simulink model "LKAS_AutoSave_DF_20220421_1805_SW62"  (R2018b)
settings: Solver=FixedStepDiscrete  StartTime=0.0  StopTime=10.0  FixedStep=0.01  RelTol=1e-3
model workspace (MAT data in the model file):
  MCOS : class17 (value not decoded)
  MCOS : class17 (value not decoded)
  MCOS : class17 (value not decoded)
  MCOS : class17 (value not decoded)
  MCOS : class17 (value not decoded)
  MCOS : class17 (value not decoded)
  MCOS : class17 (value not decoded)
  MCOS : class17 (value not decoded)
  MCOS : class17 (value not decoded)
  MCOS : class17 (value not decoded)
  MCOS : class17 (value not decoded)
  MCOS : class17 (value not decoded)
  MCOS : class17 (value not decoded)
  MCOS : class17 (value not decoded)
  MCOS : class17 (value not decoded)
  MCOS : class17 (value not decoded)
  MCOS : class17 (value not decoded)
  MCOS : class17 (value not decoded)
  MCOS : class17 (value not decoded)
  MCOS : class17 (value not decoded)
  MCOS : class17 (value not decoded)
  MCOS : class17 (value not decoded)
  MCOS : class17 (value not decoded)
  MCOS : class17 (value not decoded)
  MCOS : class17 (value not decoded)
  MCOS : class17 (value not decoded)
  MCOS : class17 (value not decoded)
  MCOS : class17 (value not decoded)
  MCOS : class17 (value not decoded)
  MCOS : class17 (value not decoded)
  MCOS : class17 (value not decoded)
  MCOS : class17 (value not decoded)
  MCOS : class17 (value not decoded)
  MCOS : class17 (value not decoded)
  MCOS : class17 (value not decoded)
  MCOS : class17 (value not decoded)
  MCOS : class17 (value not decoded)
  MCOS : class17 (value not decoded)
  MCOS : class17 (value not decoded)
  MCOS : class17 (value not decoded)
  MCOS : class17 (value not decoded)
  MCOS : class17 (value not decoded)
  MCOS : class17 (value not decoded)
  MCOS : class17 (value not decoded)
  MCOS : class17 (value not decoded)
  MCOS : class17 (value not decoded)
  MCOS : class17 (value not decoded)
  MCOS : class17 (value not decoded)
  MCOS : class17 (value not decoded)
  MCOS : class17 (value not decoded)
  MCOS : class17 (value not decoded)
  MCOS : class17 (value not decoded)
  MCOS : class17 (value not decoded)
  MCOS : class17 (value not decoded)
  MCOS : class17 (value not decoded)
  MCOS : class17 (value not decoded)
  MCOS : class17 (value not decoded)
  MCOS : class17 (value not decoded)
  MCOS : class17 (value not decoded)
  MCOS : class17 (value not decoded)
  MCOS : class17 (value not decoded)
  MCOS : class17 (value not decoded)
  MCOS : class17 (value not decoded)
  MCOS : class17 (value not decoded)
  MCOS : class17 (value not decoded)
  MCOS : class17 (value not decoded)
  MCOS : class17 (value not decoded)
  MCOS : class17 (value not decoded)
  MCOS : class17 (value not decoded)
  MCOS : class17 (value not decoded)
  MCOS : class17 (value not decoded)
  MCOS : class17 (value not decoded)
  MCOS : class17 (value not decoded)
  MCOS : class17 (value not decoded)
  MCOS : class17 (value not decoded)
  MCOS : class17 (value not decoded)
  MCOS : class17 (value not decoded)
  MCOS : class17 (value not decoded)
  MCOS : class17 (value not decoded)
  MCOS : class17 (value not decoded)
  MCOS : class17 (value not decoded)
  MCOS : class17 (value not decoded)
  MCOS : class17 (value not decoded)
  MCOS : class17 (value not decoded)
  MCOS : class17 (value not decoded)
  MCOS : class17 (value not decoded)
  MCOS : class17 (value not decoded)
  MCOS : class17 (value not decoded)
  MCOS : class17 (value not decoded)
  MCOS : class17 (value not decoded)
  MCOS : class17 (value not decoded)
  MCOS : class17 (value not decoded)
  MCOS : class17 (value not decoded)
  MCOS : class17 (value not decoded)
  MCOS : class17 (value not decoded)
  MCOS : class17 (value not decoded)
  MCOS : class17 (value not decoded)
  MCOS : class17 (value not decoded)
  MCOS : class17 (value not decoded)
  MCOS : class17 (value not decoded)
  MCOS : class17 (value not decoded)
  MCOS : class17 (value not decoded)
  MCOS : class17 (value not decoded)
  MCOS : class17 (value not decoded)
  MCOS : class17 (value not decoded)
  MCOS : class17 (value not decoded)
  MCOS : class17 (value not decoded)
  MCOS : class17 (value not decoded)
  MCOS : class17 (value not decoded)
  MCOS : class17 (value not decoded)
undefined symbols (not defined in the file): LKA_CarWidth, LKA_SampleTime, LKA_StrRatio_C, LKA_Veh2CamL_C, LKA_Veh2CamW_C, LKA_WhlBaseL_C, LL_CompHdAg_C, LL_CompSWA_C, LL_CrvtPrvwT_C, LL_DesDvt_C, LL_DvtComp_C, LL_DvtPrvwT_C, LL_DvtSpdDet_vDvtSpdMin_C, LL_HandsOff_ExitTime, LL_HandsOff_TextTime, LL_HandsOff_WarnTime, LL_HdAgExT_C, LL_HdAgPrvwT_C, LL_LAccMax_C, LL_LAccRMax_C, LL_LDW_EarliestWarnLine_C, LL_LDW_LatestWarnLine_C, LL_LDWS_SUPPRESS_HEADING, LL_LFClb_TFC_FfCtlRatio_C, LL_LFClb_TFC_KdBalance_C, LL_LFClb_TFC_KdMaxSWA_C, LL_LFClb_TFC_KdV1_C, LL_LFClb_TFC_KdV2_C, LL_LFClb_TFC_KdVehSpdLwr_C, LL_LFClb_TFC_KdVehSpdUpr_C, LL_LFClb_TFC_Ki_C, LL_LFClb_TFC_KiMaxSWA_C, LL_LFClb_TFC_Kp_C, LL_LFClb_TFC_KpKlat_C, LL_LFClb_TFC_KpV1_C, LL_LFClb_TFC_KpV2_C, LL_LFClb_TFC_KpVehSpdLwr_C, LL_LFClb_TFC_KpVehSpdUpr_C, LL_LFClb_TFC_PrvwT_C, LL_LKA_EarliestWarnLine_C, LL_LKA_EnableLine_DvtMax, LL_LKA_EnableLine_DvtMin, LL_LKA_EnableLine_Max, LL_LKA_LatestWarnLine_C, LL_LKAExPrcs_ExitC0Dvt, LL_LKAExPrcs_ExitC0Swt, LL_LKAExPrcs_tiExitDelayTime3, LL_LKAExPrcs_tiExitTime1, LL_LKAExPrcs_tiExitTime2, LL_LKAExPrcs_tiExitTime3, LL_LKAS_OUT_OF_CONTROL_LAT_VEL, LL_LKAS_OUT_OF_CONTROL_TTLC, LL_LKASWASyn_M0, LL_LKASWASyn_M1, LL_LKASWASyn_M2, LL_LKASWASyn_M3D, LL_LKASWASyn_M3K_DT, LL_LKASWASyn_M3K_MSD, LL_LKASWASyn_M4K, LL_LKASWASyn_SWAaddMax ... (+51)
libraries: simulink x241, canmsglib x6, dspstat3 x3, simulink_extras x1
(part 6 of 18)

== system LKAS_AutoSave_DF_20220421_1805_SW62/LKAS/LL/LLOn/LKA Input Processing (LKAInP) ==
  bsInInfo : Inport
  bsLLClb : Inport  Port=2
  ActFlg : Inport  Port=3
  Bus Creator2 : BusCreator  Inputs=10
  Curvature Calculation (Crvt) : Subsystem
  Delay : Delay  DelayLength=1
  Deviation Calculation (Dvt) : Subsystem
  Heading Angle Calculation (HdAg) : Subsystem
  Lane Width Calculation (LW) : Subsystem
  Previewed Curvature Calculation (PrCrvt) : Subsystem
  Previewed Deviation Calculation (PrDvt) : Subsystem
  Previewed Heading Angle Calculation (PrHdAg) : Subsystem
  Steering Wheel Position Calculation (SWAPosCal) : Subsystem
  TTLC Calculation (TTLCCalc) : Subsystem  Description=|
      | Block Name: TTLC Calculation
      | Ab.: TTLCCalc
      | No.: 1.1.1.1
      | Rev: 0.0.1
      | Update Date: 19-3-26
  Under The Limit (UndrLim) : Subsystem
  bsLKAInPInfo : Outport
  wires:
  [bsTTLCInfo] -> Previewed Heading Angle Calculation (PrHdAg)/3(PrHdAg_bsTTLCInfo)  "bsTTLCInfo"
  TTLC Calculation (TTLCCalc)/1(TTLCCalc_bsTTLCInfo) -> [bsTTLCInfo]  "bsTTLCInfo"
  Previewed Deviation Calculation (PrDvt)/1(PrvwDvt_bsPrvwDvtInfo) -> [bsPrDvtInfo]  "bsPrDvtInfo"
  Previewed Heading Angle Calculation (PrHdAg)/1(PrHdAg_bsPrHdAgInfo) -> [bsPrHdAgInfo]  "bsPrHdAgInfo"
  [bsPrCrvtInfo] -> TTLC Calculation (TTLCCalc)/4(TTLCCalc_bsPrCrvtInfo)  "bsPrCrvtInfo"
  Previewed Curvature Calculation (PrCrvt)/1(PrvwCrvt_bsPrvwCrvtInfo) -> [bsPrCrvtInfo]  "bsPrCrvtInfo"
  [bsDvtInfo] -> TTLC Calculation (TTLCCalc)/1(TTLCCalc_bsDvtInfo)  "bsDvtInfo"
  Deviation Calculation (Dvt)/1(Dvt_bsDvtInfo) -> [bsDvtInfo]  "bsDvtInfo"
  [bsHdAgInfo] -> TTLC Calculation (TTLCCalc)/5(TTLCCalc_bsHdAgInfo)  "bsHdAgInfo"
  Heading Angle Calculation (HdAg)/1(HdAg_bsHdAgInfo) -> [bsHdAgInfo]  "bsHdAgInfo"
  Curvature Calculation (Crvt)/1(Crvt_bsCrvtInfo) -> [bsCrvtInfo]  "bsCrvtInfo"
  Under The Limit (UndrLim)/1(UndrLim_bsUndrLimInfo) -> [bsUndrLimInfo]  "bsUndrLimInfo"
  Steering Wheel Position Calculation (SWAPosCal)/1(SWAPosCal) -> [phiSWAPos]  "phiSWAPos"
  Lane Width Calculation (LW)/1(LW_LaneWidth) -> [LaneWidth]  "LaneWidth"
  Delay/1 -> Previewed Curvature Calculation (PrCrvt)/3(PrvwCrvt_stLKAActvFlg)
  ActFlg/1 -> Delay/1
  Bus Creator2/1 -> bsLKAInPInfo/1
  [bsPrCrvtInfo] -> Bus Creator2/7  "bsPrCrvtInfo"
  [bsPrDvtInfo] -> Bus Creator2/9  "bsPrDvtInfo"
  [bsCrvtInfo] -> Bus Creator2/4  "bsCrvtInfo"
  [bsDvtInfo] -> Bus Creator2/6  "bsDvtInfo"
  [bsUndrLimInfo] -> Bus Creator2/3  "bsUndrLimInfo"
  [phiSWAPos] -> Bus Creator2/2  "phiSWAPos"
  [LaneWidth] -> Bus Creator2/1  "LaneWidth"
  [bsTTLCInfo] -> Bus Creator2/10  "bsTTLCInfo"
  [bsPrHdAgInfo] -> Bus Creator2/8  "bsPrHdAgInfo"
  bsLLClb/1 -> TTLC Calculation (TTLCCalc)/2(TTLCCalc_bsLLClb), Previewed Curvature Calculation (PrCrvt)/2(PrvwCrvt_tiCrvtPrvwT_C), Steering Wheel Position Calculation (SWAPosCal)/2(SWAPosCal_bsLLClb), Under The Limit (UndrLim)/2(UndrLim_bsLLClb), Deviation Calculation (Dvt)/2(Dvt_bsLLClb), Previewed Heading Angle Calculation (PrHdAg)/2(PrHdAg_bsLLClb), Previewed Deviation Calculation (PrDvt)/1(PrdcDvt_bsLLClb)
  [bsHdAgInfo] -> Bus Creator2/5  "bsHdAgInfo"
  bsInInfo/1 -> Steering Wheel Position Calculation (SWAPosCal)/1(SWAPosCal_bsInInfoSyn), Lane Width Calculation (LW)/1(LW_bsInInfoSyn), Under The Limit (UndrLim)/1(UndrLim_bsInInfoSyn), Curvature Calculation (Crvt)/1(PrvwCrvt_bsInInfoSyn), Heading Angle Calculation (HdAg)/1(HdAg_bsInInfoSyn), Deviation Calculation (Dvt)/1(Dvt_bsInInfoSyn), Previewed Curvature Calculation (PrCrvt)/1(PrvwCrvt_bsInInfoSyn), Previewed Deviation Calculation (PrDvt)/2(PrvwDvt_bsInInfoSyn), TTLC Calculation (TTLCCalc)/3(TTLCCalc_bsInfo), Previewed Heading Angle Calculation (PrHdAg)/1(PrHdAg_bsInInfoSyn)

== system LKAS_AutoSave_DF_20220421_1805_SW62/LKAS/LL/LLOn/LL State Determination (LLStateDet) ==
  bsInInfo : Inport
  bsLKAInPInfo : Inport  Port=2
  bsLLClb : Inport  Port=3
  ExitFlg : Inport  Port=4
  bsSignalFault : Inport  Port=5
  Bus Creator : BusCreator  Inputs=3
  Delay : Delay  DelayLength=1
  Delay1 : Delay  DelayLength=1
  LDW_State_Machine : Stateflow chart  Description=|  TreatAsAtomicUnit=on
      | Block Name: LDW State Machine
      | Ab.: LDWSM
      | No.: 1.1.2.0
      | Rev: 0.0.1
      | Update Date: 19-3-26
      settings: RTWSystemCode=Nonreusable function
  LKA_State_Machine : Stateflow chart  Description=|  TreatAsAtomicUnit=on
      | Block Name: LKA State Machine
      | Ab.: LKASM
      | No.: 1.1.3.0
      | Rev: 0.0.1
      | Update Date: 19-3-26
      settings: RTWSystemCode=Nonreusable function
  LL State Machine Conditions (LLSMCon) : Subsystem
  bsLLState : Outport
  stLDWActvFlg : Outport  Port=2
  stLKAActvFlg : Outport  Port=3
  Disable_Reason : Outport  Port=4
  Fault_Reason : Outport  Port=5
  tag scope: LDW_State_Mon=global, LKA_State_Mon=global
  wires:
  [LKA_Mode] -> Bus Creator/2
  [LKA_Mode] -> LKA_State_Machine/1(LKA_Mode)
  [LKA_Mode] -> LDW_State_Machine/1(LKA_Mode)
  LL State Machine Conditions (LLSMCon)/1(LKA_Mode) -> [LKA_Mode]  "LKA_Mode"
  LL State Machine Conditions (LLSMCon)/13(Fault_Reason) -> Fault_Reason/1
  LL State Machine Conditions (LLSMCon)/12(Disable_Reason) -> Disable_Reason/1
  bsSignalFault/1 -> LL State Machine Conditions (LLSMCon)/6(bsSignalFault)
  Delay/1 -> LL State Machine Conditions (LLSMCon)/5(ExitFlg)
  bsLLClb/1 -> LL State Machine Conditions (LLSMCon)/3(bsLLClb)
  ExitFlg/1 -> Delay/1
  bsLKAInPInfo/1 -> LL State Machine Conditions (LLSMCon)/2(bsLKAInPInfo)
  bsInInfo/1 -> LL State Machine Conditions (LLSMCon)/1(bsInInfo)
  LL State Machine Conditions (LLSMCon)/11(LKA_Fault) -> LKA_State_Machine/6(LKA_Fault)
  LL State Machine Conditions (LLSMCon)/10(stLKADeactvCSyn) -> LKA_State_Machine/5(stLKADeactvCSyn)
  LL State Machine Conditions (LLSMCon)/9(stLKAActvCSyn) -> LKA_State_Machine/4(stLKAActvCSyn)
  LL State Machine Conditions (LLSMCon)/8(stLKADisblCSyn) -> LKA_State_Machine/3(stLKADisblCSyn)
  LL State Machine Conditions (LLSMCon)/7(stLKAEnaCSyn) -> LKA_State_Machine/2(stLKAEnaCSyn)
  LL State Machine Conditions (LLSMCon)/6(LDW_Fault) -> LDW_State_Machine/6(LDW_Fault)
  LDW_State_Machine/2(stLDWState) -> Bus Creator/1, [LDW_State_Mon]  "LDW_State"
  LKA_State_Machine/2(stLKAState) -> [LKA_State_Mon], Bus Creator/3  "LKA_State"
  Bus Creator/1 -> Delay1/1, bsLLState/1  "bsLLState"
  Delay1/1 -> LL State Machine Conditions (LLSMCon)/4(bsLLState)
  LKA_State_Machine/1(stLKAActvFlg) -> stLKAActvFlg/1
  LDW_State_Machine/1(stLDWActvFlg) -> stLDWActvFlg/1
  LL State Machine Conditions (LLSMCon)/5(stLDWDeactvCSyn) -> LDW_State_Machine/5(stLDWDeactvCSyn)  "stLDWDeactvCSyn"
  LL State Machine Conditions (LLSMCon)/4(stLDWActvCSyn) -> LDW_State_Machine/4(stLDWActvCSyn)
  LL State Machine Conditions (LLSMCon)/3(stLDWDisblCSyn) -> LDW_State_Machine/3(stLDWDisblCSyn)
  LL State Machine Conditions (LLSMCon)/2(stLDWEnaCSyn) -> LDW_State_Machine/2(stLDWEnaCSyn)

== system LKAS_AutoSave_DF_20220421_1805_SW62/LKAS/LL/LLOn/LL_Mon ==
  Disable_Reason : Inport
  Fault_Reason : Inport  Port=2
  LKAMon : Inport  Port=3
  Bus : BusCreator  Inputs=5
  BusInP : BusCreator  Inputs=2
  BusState : BusCreator  Inputs=2
  LLMon : Outport
  wires:
  Fault_Reason/1 -> Bus/5  "Fault_Reason"
  Disable_Reason/1 -> Bus/4  "Disable_Reason"
  BusState/1 -> [StateMon]  "StateMon"
  BusInP/1 -> [InPMon]  "InPMon"
  [LKA_State_Mon] -> BusState/2  "LKA_State_Mon"
  [LDW_State_Mon] -> BusState/1  "LDW_State_Mon"
  [RGTTTLC_Mon] -> BusInP/2  "RGTTTLC_Mon"
  [LFTTTLC_Mon] -> BusInP/1  "LFTTTLC_Mon"
  Bus/1 -> LLMon/1  "LLMon"
  LKAMon/1 -> Bus/3
  [StateMon] -> Bus/2
  [InPMon] -> Bus/1

== system LKAS_AutoSave_DF_20220421_1805_SW62/LKAS/LL/LLOut/Angle2Trq ==
  LKA_Torque_Req : Inport
  Target_Angle : Inport  Port=2
  Stearing_Angle : Inport  Port=3
  Constant : Constant  Value=5  OutDataTypeStr=single
  Constant1 : Constant  Value=-5  OutDataTypeStr=single
  Constant3 : Constant  Value=5  OutDataTypeStr=single
  Constant4 : Constant  Value=-5  OutDataTypeStr=single
  Rate Limiter Dynamic : Subsystem
  Saturation Dynamic : Subsystem
  Subsystem : Subsystem
  torque : Outport  OutputWhenDisabled=reset  InitialOutput=0
  wires:
  LKA_Torque_Req/1 -> Subsystem/Enable  "LKA_Torque_Req"
  Subsystem/1(in_trq) -> Rate Limiter Dynamic/2(u)  "in_trq"
  Stearing_Angle/1 -> Subsystem/2(Stearing_Angle)  "Stearing_Angle"
  Target_Angle/1 -> Subsystem/1(Target_Angle)  "Target_Angle"
  Constant/1 -> Rate Limiter Dynamic/1(up)
  Constant1/1 -> Rate Limiter Dynamic/3(lo)
  Rate Limiter Dynamic/1(Y) -> Saturation Dynamic/2(u)  "RL_trq"
  Constant3/1 -> Saturation Dynamic/1(up)
  Constant4/1 -> Saturation Dynamic/3(lo)
  Saturation Dynamic/1(y) -> torque/1  "Saturation_trq"

== system LKAS_AutoSave_DF_20220421_1805_SW62/LKAS/LLClb/LLSMConClb/ICv to v10 ==
  In1 : Inport
  Add : Sum  Inputs=+-
  Constant : Constant  Value=2.5  OutDataTypeStr=single
  Gain : Gain  Gain=1/1.02
  Out1 : Outport
  wires:
  Gain/1 -> Out1/1
  Constant/1 -> Add/2
  Add/1 -> Gain/1
  In1/1 -> Add/1

== system LKAS_AutoSave_DF_20220421_1805_SW62/LKAS/LLClb/LLSMConClb/ICv to v11 ==
  In1 : Inport
  Add : Sum  Inputs=+-
  Constant : Constant  Value=2.5  OutDataTypeStr=single
  Gain : Gain  Gain=1/1.02
  Out1 : Outport
  wires:
  In1/1 -> Add/1
  Add/1 -> Gain/1
  Constant/1 -> Add/2
  Gain/1 -> Out1/1

== system LKAS_AutoSave_DF_20220421_1805_SW62/LKAS/LLClb/LLSMConClb/ICv to v6 ==
  In1 : Inport
  Add : Sum  Inputs=+-
  Constant : Constant  Value=2.5  OutDataTypeStr=single
  Gain : Gain  Gain=1/1.02
  Out1 : Outport
  wires:
  Gain/1 -> Out1/1
  Constant/1 -> Add/2
  Add/1 -> Gain/1
  In1/1 -> Add/1

== system LKAS_AutoSave_DF_20220421_1805_SW62/LKAS/LLClb/LLSMConClb/ICv to v7 ==
  In1 : Inport
  Add : Sum  Inputs=+-
  Constant : Constant  Value=2.5  OutDataTypeStr=single
  Gain : Gain  Gain=1/1.02
  Out1 : Outport
  wires:
  In1/1 -> Add/1
  Add/1 -> Gain/1
  Constant/1 -> Add/2
  Gain/1 -> Out1/1

== system LKAS_AutoSave_DF_20220421_1805_SW62/LKAS/LLClb/LLSMConClb/ICv to v8 ==
  In1 : Inport
  Add : Sum  Inputs=+-
  Constant : Constant  Value=2.5  OutDataTypeStr=single
  Gain : Gain  Gain=1/1.02
  Out1 : Outport
  wires:
  Gain/1 -> Out1/1
  Constant/1 -> Add/2
  Add/1 -> Gain/1
  In1/1 -> Add/1

== system LKAS_AutoSave_DF_20220421_1805_SW62/LKAS/LLClb/LLSMConClb/ICv to v9 ==
  In1 : Inport
  Add : Sum  Inputs=+-
  Constant : Constant  Value=2.5  OutDataTypeStr=single
  Gain : Gain  Gain=1/1.02
  Out1 : Outport
  wires:
  In1/1 -> Add/1
  Add/1 -> Gain/1
  Constant/1 -> Add/2
  Gain/1 -> Out1/1

== system LKAS_AutoSave_DF_20220421_1805_SW62/LKAS/LL/Human Machine Interface (HMI)/Subsystem/Sum Condition1 ==
  SampleTime : Inport
  Sum : Inport  Port=2
  state = reset : EnablePort  StatesWhenEnabling=reset
  Add1 : Sum  OutDataTypeStr=single
  Memory : Memory  InheritSampleTime=on
  Relational Operator : RelationalOperator  OutDataTypeStr=boolean  RndMeth=Nearest
  Saturation : Saturate  UpperLimit=60  LowerLimit=0
      settings: AttributesFormatString="Min = %<LowerLimit>  Max = %<UpperLimit>"
  Out : Outport  OutputWhenDisabled=reset  InitialOutput=0
      settings: AttributesFormatString=%<OutputWhenDisabled> = %<InitialOutput>
  wires:
  SampleTime/1 -> Add1/1
  Saturation/1 -> Relational Operator/1, Memory/1
  Relational Operator/1 -> Out/1
  Sum/1 -> Relational Operator/2
  Add1/1 -> Saturation/1
  Memory/1 -> Add1/2

== system LKAS_AutoSave_DF_20220421_1805_SW62/LKAS/LL/Human Machine Interface (HMI)/Subsystem/Sum Condition2 ==
  SampleTime : Inport
  Sum : Inport  Port=2
  state = reset : EnablePort  StatesWhenEnabling=reset
  Add1 : Sum  OutDataTypeStr=single
  Memory : Memory  InheritSampleTime=on
  Relational Operator : RelationalOperator  OutDataTypeStr=boolean  RndMeth=Nearest
  Saturation : Saturate  UpperLimit=60  LowerLimit=0
      settings: AttributesFormatString="Min = %<LowerLimit>  Max = %<UpperLimit>"
  Out : Outport  OutputWhenDisabled=reset  InitialOutput=0
      settings: AttributesFormatString=%<OutputWhenDisabled> = %<InitialOutput>
  wires:
  Memory/1 -> Add1/2
  Add1/1 -> Saturation/1
  Sum/1 -> Relational Operator/2
  Relational Operator/1 -> Out/1
  Saturation/1 -> Memory/1, Relational Operator/1
  SampleTime/1 -> Add1/1

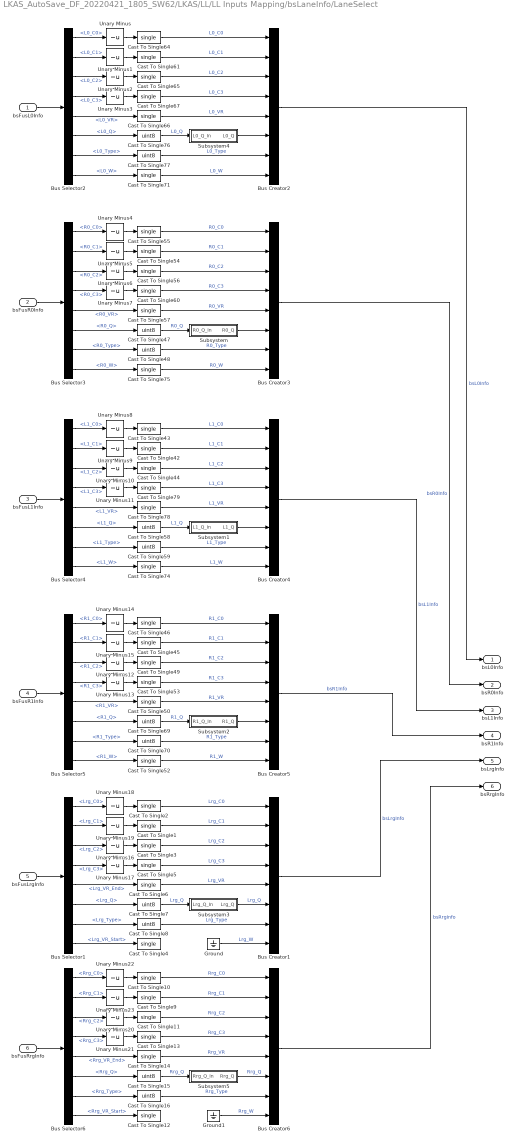
== system LKAS_AutoSave_DF_20220421_1805_SW62/LKAS/LL/LL Inputs Mapping/bsLaneInfo/LaneSelect ==
  bsFusL0Info : Inport
  bsFusR0Info : Inport  Port=2
  bsFusL1Info : Inport  Port=3
  bsFusR1Info : Inport  Port=4
  bsFusLrgInfo : Inport  Port=5
  bsFusRrgInfo : Inport  Port=6
  Bus Creator{1..6} (6 alike) : BusCreator  Inputs=8
  Bus Selector1 : BusSelector  OutputSignals=Lrg_C0,Lrg_C1,Lrg_C2,Lrg_C3,Lrg_VR_End,Lrg_Q,Lrg_Type,Lrg_VR_Start
  Bus Selector2 : BusSelector  OutputSignals=L0_C0,L0_C1,L0_C2,L0_C3,L0_VR,L0_Q,L0_Type,L0_W
  Bus Selector3 : BusSelector  OutputSignals=R0_C0,R0_C1,R0_C2,R0_C3,R0_VR,R0_Q,R0_Type,R0_W
  Bus Selector4 : BusSelector  OutputSignals=L1_C0,L1_C1,L1_C2,L1_C3,L1_VR,L1_Q,L1_Type,L1_W
  Bus Selector5 : BusSelector  OutputSignals=R1_C0,R1_C1,R1_C2,R1_C3,R1_VR,R1_Q,R1_Type,R1_W
  Bus Selector6 : BusSelector  OutputSignals=Rrg_C0,Rrg_C1,Rrg_C2,Rrg_C3,Rrg_VR_End,Rrg_Q,Rrg_Type,Rrg_VR_Start
  Cast To Single{1..6,9..14,42..46,49..50,52..57,60..61,64..67,71,74..75,78..79} (36 alike) : DataTypeConversion  OutDataTypeStr=single
  Cast To Single{7..8,15..16,47..48,58..59,69..70,76..77} (12 alike) : DataTypeConversion  OutDataTypeStr=uint8
  Ground : Ground
  Ground1 : Ground
  Subsystem : Subsystem
  Subsystem1 : Subsystem
  Subsystem2 : Subsystem
  Subsystem3 : Subsystem
  Subsystem4 : Subsystem
  Subsystem5 : Subsystem
  Unary Minus{,1..23} (24 alike) : UnaryMinus
  bsL0Info : Outport
  bsR0Info : Outport  Port=2
  bsL1Info : Outport  Port=3
  bsR1Info : Outport  Port=4
  bsLrgInfo : Outport  Port=5
  bsRrgInfo : Outport  Port=6
  wires:
  Subsystem5/1(Rrg_Q) -> Bus Creator6/6  "Rrg_Q"
  Subsystem3/1(Lrg_Q) -> Bus Creator1/6  "Lrg_Q"
  Unary Minus23/1 -> Cast To Single9/1
  Unary Minus22/1 -> Cast To Single10/1
  Unary Minus21/1 -> Cast To Single13/1
  Unary Minus20/1 -> Cast To Single11/1
  Unary Minus17/1 -> Cast To Single5/1
  Unary Minus19/1 -> Cast To Single1/1
  Unary Minus18/1 -> Cast To Single2/1
  Unary Minus16/1 -> Cast To Single3/1
  Bus Creator6/1 -> bsRrgInfo/1  "bsRrgInfo"
  Bus Creator1/1 -> bsLrgInfo/1  "bsLrgInfo"
  Ground1/1 -> Bus Creator6/8  "Rrg_W"
  Cast To Single16/1 -> Bus Creator6/7  "Rrg_Type"
  Cast To Single15/1 -> Subsystem5/1(Rrg_Q_In)  "Rrg_Q"
  Cast To Single14/1 -> Bus Creator6/5  "Rrg_VR"
  Cast To Single13/1 -> Bus Creator6/4  "Rrg_C3"
  Cast To Single11/1 -> Bus Creator6/3  "Rrg_C2"
  Cast To Single9/1 -> Bus Creator6/2  "Rrg_C1"
  Cast To Single10/1 -> Bus Creator6/1  "Rrg_C0"
  Bus Selector6/7 -> Cast To Single16/1  "<Rrg_Type>"
  Bus Selector6/6 -> Cast To Single15/1  "<Rrg_Q>"
  Bus Selector6/5 -> Cast To Single14/1  "<Rrg_VR_End>"
  Bus Selector6/8 -> Cast To Single12/1  "<Rrg_VR_Start>"
  Bus Selector6/4 -> Unary Minus21/1  "<Rrg_C3>"
  Bus Selector6/3 -> Unary Minus20/1  "<Rrg_C2>"
  Bus Selector6/2 -> Unary Minus23/1  "<Rrg_C1>"
  Bus Selector6/1 -> Unary Minus22/1  "<Rrg_C0>"
  Ground/1 -> Bus Creator1/8  "Lrg_W"
  Cast To Single8/1 -> Bus Creator1/7  "Lrg_Type"
  Cast To Single7/1 -> Subsystem3/1(Lrg_Q_In)  "Lrg_Q"
  Cast To Single5/1 -> Bus Creator1/4  "Lrg_C3"
  Cast To Single6/1 -> Bus Creator1/5  "Lrg_VR"
  Cast To Single2/1 -> Bus Creator1/1  "Lrg_C0"
  Cast To Single3/1 -> Bus Creator1/3  "Lrg_C2"
  Cast To Single1/1 -> Bus Creator1/2  "Lrg_C1"
  Bus Selector1/7 -> Cast To Single8/1  "<Lrg_Type>"
  Bus Selector1/6 -> Cast To Single7/1  "<Lrg_Q>"
  Bus Selector1/5 -> Cast To Single6/1  "<Lrg_VR_End>"
  Bus Selector1/8 -> Cast To Single4/1  "<Lrg_VR_Start>"
  Bus Selector1/4 -> Unary Minus17/1  "<Lrg_C3>"
  Bus Selector1/3 -> Unary Minus16/1  "<Lrg_C2>"
  Bus Selector1/2 -> Unary Minus19/1  "<Lrg_C1>"
  Bus Selector1/1 -> Unary Minus18/1  "<Lrg_C0>"
  bsFusRrgInfo/1 -> Bus Selector6/1
  bsFusLrgInfo/1 -> Bus Selector1/1
  Subsystem2/1(R1_Q) -> Bus Creator5/6
  Subsystem1/1(L1_Q) -> Bus Creator4/6
  Unary Minus15/1 -> Cast To Single45/1
  Unary Minus14/1 -> Cast To Single46/1
  Unary Minus13/1 -> Cast To Single53/1
  Unary Minus12/1 -> Cast To Single49/1
  Unary Minus10/1 -> Cast To Single44/1
  Unary Minus11/1 -> Cast To Single79/1
  Unary Minus9/1 -> Cast To Single42/1
  Unary Minus8/1 -> Cast To Single43/1
  Unary Minus5/1 -> Cast To Single54/1
  Unary Minus4/1 -> Cast To Single55/1
  Unary Minus6/1 -> Cast To Single56/1
  Unary Minus7/1 -> Cast To Single60/1
  Unary Minus3/1 -> Cast To Single67/1
  Unary Minus2/1 -> Cast To Single65/1
  Unary Minus1/1 -> Cast To Single61/1
  Unary Minus/1 -> Cast To Single64/1
  Cast To Single71/1 -> Bus Creator2/8  "L0_W"
  Cast To Single70/1 -> Bus Creator5/7  "R1_Type"
  Cast To Single69/1 -> Subsystem2/1(R1_Q_In)  "R1_Q"
  Cast To Single53/1 -> Bus Creator5/4  "R1_C3"
  Cast To Single52/1 -> Bus Creator5/8  "R1_W"
  Cast To Single50/1 -> Bus Creator5/5  "R1_VR"
  Cast To Single49/1 -> Bus Creator5/3  "R1_C2"
  Cast To Single46/1 -> Bus Creator5/1  "R1_C0"
  Cast To Single45/1 -> Bus Creator5/2  "R1_C1"
  Cast To Single74/1 -> Bus Creator4/8  "L1_W"
  Cast To Single79/1 -> Bus Creator4/4  "L1_C3"
  Cast To Single78/1 -> Bus Creator4/5  "L1_VR"
  Cast To Single42/1 -> Bus Creator4/2  "L1_C1"
  Cast To Single43/1 -> Bus Creator4/1  "L1_C0"
  Cast To Single59/1 -> Bus Creator4/7  "L1_Type"
  Cast To Single58/1 -> Subsystem1/1(L1_Q_In)  "L1_Q"
  Cast To Single44/1 -> Bus Creator4/3  "L1_C2"
  Cast To Single75/1 -> Bus Creator3/8  "R0_W"
  Cast To Single60/1 -> Bus Creator3/4  "R0_C3"
  Cast To Single57/1 -> Bus Creator3/5  "R0_VR"
  Cast To Single48/1 -> Bus Creator3/7  "R0_Type"
  Cast To Single47/1 -> Subsystem/1(R0_Q_In)  "R0_Q"
  Cast To Single55/1 -> Bus Creator3/1  "R0_C0"
  Cast To Single54/1 -> Bus Creator3/2  "R0_C1"
  Cast To Single56/1 -> Bus Creator3/3  "R0_C2"
  Cast To Single77/1 -> Bus Creator2/7  "L0_Type"
  Cast To Single76/1 -> Subsystem4/1(L0_Q_In)  "L0_Q"
  Cast To Single64/1 -> Bus Creator2/1  "L0_C0"
  Cast To Single65/1 -> Bus Creator2/3  "L0_C2"
  Cast To Single67/1 -> Bus Creator2/4  "L0_C3"
  Cast To Single66/1 -> Bus Creator2/5  "L0_VR"
  Cast To Single61/1 -> Bus Creator2/2  "L0_C1"
  Bus Creator2/1 -> bsL0Info/1  "bsL0Info"
  Bus Creator3/1 -> bsR0Info/1  "bsR0Info"
  Bus Creator4/1 -> bsL1Info/1  "bsL1Info"
  Bus Selector4/5 -> Cast To Single78/1  "<L1_VR>"
  Bus Selector4/2 -> Unary Minus9/1  "<L1_C1>"
  Bus Selector3/5 -> Cast To Single57/1  "<R0_VR>"
  Subsystem4/1(L0_Q) -> Bus Creator2/6
  Bus Selector4/1 -> Unary Minus8/1  "<L1_C0>"
  Bus Selector2/4 -> Unary Minus3/1  "<L0_C3>"
  Bus Selector2/6 -> Cast To Single76/1  "<L0_Q>"
  bsFusR1Info/1 -> Bus Selector5/1
  bsFusL1Info/1 -> Bus Selector4/1
  bsFusR0Info/1 -> Bus Selector3/1
  Bus Selector4/7 -> Cast To Single59/1  "<L1_Type>"
  bsFusL0Info/1 -> Bus Selector2/1
  Bus Selector2/3 -> Unary Minus2/1  "<L0_C2>"
  Bus Selector5/1 -> Unary Minus14/1  "<R1_C0>"
  Bus Selector3/8 -> Cast To Single75/1  "<R0_W>"
  Bus Selector3/7 -> Cast To Single48/1  "<R0_Type>"
  Bus Selector3/3 -> Unary Minus6/1  "<R0_C2>"
  Bus Selector5/7 -> Cast To Single70/1  "<R1_Type>"
  Bus Selector5/6 -> Cast To Single69/1  "<R1_Q>"
  Bus Selector5/5 -> Cast To Single50/1  "<R1_VR>"
  Bus Selector2/5 -> Cast To Single66/1  "<L0_VR>"
  Bus Selector2/1 -> Unary Minus/1  "<L0_C0>"
  Bus Selector3/4 -> Unary Minus7/1  "<R0_C3>"
  Bus Selector2/8 -> Cast To Single71/1  "<L0_W>"
  Bus Selector3/2 -> Unary Minus5/1  "<R0_C1>"
  Bus Selector3/1 -> Unary Minus4/1  "<R0_C0>"
  Bus Selector2/2 -> Unary Minus1/1  "<L0_C1>"
  Bus Selector4/4 -> Unary Minus11/1  "<L1_C3>"
  Bus Selector4/6 -> Cast To Single58/1  "<L1_Q>"
  Bus Selector2/7 -> Cast To Single77/1  "<L0_Type>"
  Subsystem/1(R0_Q) -> Bus Creator3/6
  Bus Selector3/6 -> Cast To Single47/1  "<R0_Q>"
  Bus Selector5/4 -> Unary Minus13/1  "<R1_C3>"
  Bus Creator5/1 -> bsR1Info/1  "bsR1Info"
  Bus Selector5/8 -> Cast To Single52/1  "<R1_W>"
  Bus Selector5/2 -> Unary Minus15/1  "<R1_C1>"
  Bus Selector5/3 -> Unary Minus12/1  "<R1_C2>"
  Bus Selector4/8 -> Cast To Single74/1  "<L1_W>"
  Bus Selector4/3 -> Unary Minus10/1  "<L1_C2>"

== system LKAS_AutoSave_DF_20220421_1805_SW62/LKAS/LL/LL Inputs Mapping/bsLaneInfo/LanesReconstruct  ==
  bsLLClb : Inport
  bsL0Info : Inport  Port=2
  bsR0Info : Inport  Port=3
  bsL1Info : Inport  Port=4
  bsR1Info : Inport  Port=5
  bsLrgInfo : Inport  Port=6
  bsRrgInfo : Inport  Port=7
  Bus Selector5 : BusSelector  OutputSignals=L0_Q
  Bus Selector6 : BusSelector  OutputSignals=R0_Q
  LaneReconstructSM : Stateflow chart  TreatAsAtomicUnit=on
  Left 1Lane Reconstruct (Lft1LaneR) : Subsystem
  Left Lane Reconstruct (LftLaneR) : Subsystem
  Right 1Lane Reconstruct (Rgt1LaneR) : Subsystem
  Right Lane Reconstruct (RgtLaneR) : Subsystem
  RoadSide Offset : Subsystem
  Switch : Switch  Criteria=u2 > Threshold
  Switch1 : Switch  Criteria=u2 > Threshold
  bsL0InfoR : Outport
  bsR0InfoR : Outport  Port=2
  bsL1InfoR : Outport  Port=3
  bsR1InfoR : Outport  Port=4
  wires:
  bsRrgInfo/1 -> RoadSide Offset/4(bsRrgInfo)
  bsLrgInfo/1 -> RoadSide Offset/3(bsLrgInfo)
  bsLLClb/1 -> RoadSide Offset/5(bsLLClb)
  RoadSide Offset/2(bsR0Infoout) -> Bus Selector6/1, Left Lane Reconstruct (LftLaneR)/2(bsR0Info), Right Lane Reconstruct (RgtLaneR)/2(bsR0Info), Switch/1
  RoadSide Offset/1(bsL0Infoout) -> Bus Selector5/1, Right Lane Reconstruct (RgtLaneR)/1(bsL0Info), Switch1/1, Left Lane Reconstruct (LftLaneR)/3(bsL0Info)
  bsL0Info/1 -> RoadSide Offset/1(bsL0Info)
  bsR0Info/1 -> RoadSide Offset/2(bsR0Info)
  [LftFlg] -> Switch1/2
  [RgtFlg] -> Switch/2
  [LftFlg] -> Left 1Lane Reconstruct (Lft1LaneR)/1(stFlag)
  [RgtFlg] -> Right 1Lane Reconstruct (Rgt1LaneR)/1(stFlag)
  Left 1Lane Reconstruct (Lft1LaneR)/1(bsL1InfoR) -> bsL1InfoR/1
  Right 1Lane Reconstruct (Rgt1LaneR)/1(bsL1InfoR) -> bsR1InfoR/1
  bsR1Info/1 -> Right 1Lane Reconstruct (Rgt1LaneR)/2(bsR1Info)
  LaneReconstructSM/3(LaneRSM_stRgtFlg) -> [RgtFlg]
  LaneReconstructSM/2(LaneRSM_stLftFlg) -> [LftFlg]
  LaneReconstructSM/1(LaneRSM_stRoadFlg) -> [RoadFlg]
  Switch1/1 -> bsL0InfoR/1
  Switch/1 -> bsR0InfoR/1
  Right Lane Reconstruct (RgtLaneR)/1(bsR0InfoR) -> Switch/3
  Left Lane Reconstruct (LftLaneR)/1(bsL0InfoR) -> Switch1/3
  RoadSide Offset/3(lRoadW) -> [RoadWidth], Right Lane Reconstruct (RgtLaneR)/3(lRoadW), Left Lane Reconstruct (LftLaneR)/1(lRoadW)
  Bus Selector5/1 -> LaneReconstructSM/1(LaneRSM_stL0Ql)  "<L0_Q>"
  Bus Selector6/1 -> LaneReconstructSM/2(LaneRSM_stR0Ql)  "<R0_Q>"
  bsL1Info/1 -> Left 1Lane Reconstruct (Lft1LaneR)/2(bsL1Info)

== system LKAS_AutoSave_DF_20220421_1805_SW62/LKAS/LL/LLOn/LDW/Heading Angle Detection (HdAgDet) ==
  Enable : Inport
  phiHdAg_Lft : Inport  Port=2
  phiHdAg_Rgt : Inport  Port=3
  LL_LDWS_SUPPRESS_HEADING : Inport  Port=4
  LKA_SampleTime : Inport  Port=5
  Constant : Constant  Value=0.05  OutDataTypeStr=single
  If : If  IfExpression=u1==1  ElseIfExpressions=u1==2
  If Action Subsystem : Subsystem  TreatAsAtomicUnit=on
  If Action Subsystem1 : Subsystem  TreatAsAtomicUnit=on
  If Action Subsystem2 : Subsystem  TreatAsAtomicUnit=on
  Merge : Merge  Inputs=3  InitialOutput=0
  Relational Operator : RelationalOperator  OutDataTypeStr=boolean  RndMeth=Nearest
  Sum Condition : Subsystem
  stHdAgDetFlg : Outport
  wires:
  Sum Condition/1(Out) -> stHdAgDetFlg/1
  Constant/1 -> Sum Condition/2(Sum)
  Relational Operator/1 -> Sum Condition/Enable
  LL_LDWS_SUPPRESS_HEADING/1 -> Relational Operator/2
  Merge/1 -> Relational Operator/1
  Enable/1 -> If/1
  phiHdAg_Rgt/1 -> If Action Subsystem1/1(In1)
  phiHdAg_Lft/1 -> If Action Subsystem/1(In1)
  If/3 -> If Action Subsystem2/Action
  If Action Subsystem2/1(Out1) -> Merge/3
  If/2 -> If Action Subsystem1/Action
  If Action Subsystem1/1(Out1) -> Merge/2
  If Action Subsystem/1(Out1) -> Merge/1
  If/1 -> If Action Subsystem/Action
  LKA_SampleTime/1 -> Sum Condition/1(In)

== system LKAS_AutoSave_DF_20220421_1805_SW62/LKAS/LL/LLOn/LKA/Driver Torque Addition (DTA) ==
  DTA_bsInInfoSyn : Inport
  DTA_bsLFClb : Inport  Port=2
  DTA_Exit3Flg : Inport  Port=3
  Bus Selector : BusSelector  OutputSignals=bsLKAClb.LL_LKASWAClb.LL_LKASWASyn_TrqSwaAddSwt,bsLKAClb.LL_LKASWAClb.LL_LKASWASyn_TrqFctSwt
  Compare To Constant : simulink/Logic and Bit Operations/Compare To Constant  relop=>  const=0  OutDataTypeStr=boolean
  Driver Torque Assist : Subsystem
  Subsystem : Subsystem
  Subsystem1 : Subsystem
  Switch : Switch  Criteria=u2 > Threshold
  DTA_phiDTASWACmd : Outport
  DTA_M : Outport  Port=2
  wires:
  DTA_Exit3Flg/1 -> Driver Torque Assist/3(DTA_Exit3Flg)
  Compare To Constant/1 -> Subsystem/Enable
  Bus Selector/1 -> Compare To Constant/1  "<LL_LKASWASyn_TrqSwaAddSwt>"
  Switch/1 -> DTA_M/1
  Subsystem/1(DTA_phiDTASWACmd) -> DTA_phiDTASWACmd/1
  DTA_bsInInfoSyn/1 -> Subsystem/1(DTA_bsInInfoSyn), Subsystem1/2(Trq), Driver Torque Assist/1(DTA_bsInInfoSyn)
  DTA_bsLFClb/1 -> Subsystem/2(DTA_bsLFClb), Bus Selector/1, Driver Torque Assist/2(DTA_bsLFClb), Subsystem1/1(In1)
  Subsystem1/1(TrqFactorOut) -> Switch/3
  Bus Selector/2 -> Switch/2  "<LL_LKASWASyn_TrqFctSwt>"
  Driver Torque Assist/1(DTA_M) -> Switch/1

== system LKAS_AutoSave_DF_20220421_1805_SW62/LKAS/LL/LLOn/LKA/LKA Exit Processing (LKAExPrcs) ==
  LKAExPrcs_bsLKAInPInfo : Inport
  LKAExPrcs_bsLKAClb : Inport  Port=2
  LKAExPrcs_PlanT1 : Inport  Port=3
  Cast To Single : DataTypeConversion  OutDataTypeStr=single
  Exit Time 1 : Subsystem
  Exit Time 2 : Subsystem
  Exit Time 3 : Subsystem
  Fcn : Fcn  Expr=u(3)*(u(3)==1)*3+u(2)*(u(3)==0)*2+u(1)*(u(2)==0&&u(3)==0)
  Logical Operator3 : Logic  Operator=OR  Inputs=3  AllPortsSameDT=off  OutDataTypeStr=boolean
  Mux : Mux  Inputs=3
  LKAExPrcs_stExFlg : Outport
  LKAExPrcs_stExNum : Outport  Port=2
  LKAExPrcs_stExit3Flg : Outport  Port=3
  wires:
  Exit Time 3/2(Exit3_flg) -> LKAExPrcs_stExit3Flg/1
  Cast To Single/1 -> Fcn/1
  Fcn/1 -> LKAExPrcs_stExNum/1  "ExNum"
  Mux/1 -> Cast To Single/1
  LKAExPrcs_PlanT1/1 -> Exit Time 2/3(T1), Exit Time 3/3(T1)
  LKAExPrcs_bsLKAClb/1 -> Exit Time 3/2(bsLKAClb), Exit Time 2/1(bsLKAClb), Exit Time 1/2(bsLKAClb)
  LKAExPrcs_bsLKAInPInfo/1 -> Exit Time 1/1(bsLKAInPInfo), Exit Time 3/1(bsLKAInPInfo), Exit Time 2/2(bsLKAInPInfo)
  Exit Time 3/1(Exit3) -> Logical Operator3/3, Mux/3  "Exit3"
  Exit Time 2/1(Exit2) -> Logical Operator3/2, Mux/2  "Exit2"
  Exit Time 1/1(Exit1) -> Logical Operator3/1, Mux/1  "Exit1"
  Logical Operator3/1 -> LKAExPrcs_stExFlg/1

== system LKAS_AutoSave_DF_20220421_1805_SW62/LKAS/LL/LLOn/LKA/LKA Motion Planning (LKAMP)  ==
  LKAMP_bsInInfoSyn : Inport
  LKAMP_Ff : Inport  Port=2
  LKAMP_stLKAActvFlg : Inport  Port=3
  LKAMP_bsLKAInPInfo : Inport  Port=4
  LKAMP_bsLLClb : Inport  Port=5
  Bus Selector : BusSelector  OutputSignals=MPInP_vVehSpdIni
  Bus Selector1 : BusSelector  OutputSignals=bsVehMovInfo.ESC_VehSpd
  Bus Selector3 : BusSelector  OutputSignals=bsConstantClb.LKA_CarWidth,bsLKAClb.LL_HdAgExT_C,bsLKAClb.LL_LSpdCompT_C
  Bus Selector4 : BusSelector  OutputSignals=bsVehMovInfo.ESC_VehSpd
  Bus Selector5 : BusSelector  OutputSignals=LaneWidth
  LKA Motion Planning Calculation (LKAMPCal) : Subsystem  Description=|
      | Block Name: LKA Motion Planning Calculation
      | Ab.: LKAMPCal
      | No.: 1.2.3.2
      | Rev: 0.0.1
      | Update Date: 19-3-26
      settings: RTWSystemCode=Nonreusable function
  Motion Planning Input Processing (MPInP) : Subsystem  Description=|
      | Block Name: Motion Planning Input Processing
      | Ab.: MPInP
      | No.: 1.2.3.1
      | Rev: 0.0.1
      | Update Date: 19-3-26
  Nominal Time Calculation (NomTCalc) : Subsystem  Description=|
      | Block Name: Nominal Time Calculation
      | Ab.: NomTCalc
      | No.: 1.2.3.3
      | Rev: 0.0.1
      | Update Date: 19-3-26
  Saturation6 : Saturate  UpperLimit=2  LowerLimit=0.2
      settings: AttributesFormatString="Min = %<LowerLimit>  Max = %<UpperLimit>"
  Steering Wheel Angle Command Calculation (SWACmdCal) : Subsystem  Description=|
      | Block Name: Steering Wheel Angle Command Calculation
      | Ab.: SWACmdCal
      | No.: 1.2.3.4
      | Rev: 0.0.1
      | Update Date: 19-3-26
  Switching Condition (SwtCon) : Subsystem
  Trigger Once : Subsystem
  LKAMP_phiSWACmd : Outport
  LKAMP_tiT1 : Outport  Port=2
  wires:
  Trigger Once/1(Out1) -> LKA Motion Planning Calculation (LKAMPCal)/Action
  LKAMP_Ff/1 -> Motion Planning Input Processing (MPInP)/1(MPInP_Ff)
  Bus Selector3/1 -> Switching Condition (SwtCon)/5(SwtCon_lCarWidth_C)  "<LKA_CarWidth>"
  Bus Selector5/1 -> Switching Condition (SwtCon)/4(SwtCon_lLaneWidth_C)  "<LaneWidth>"
  Saturation6/1 -> LKAMP_tiT1/1
  LKAMP_bsInInfoSyn/1 -> Bus Selector4/1, Bus Selector1/1, Motion Planning Input Processing (MPInP)/5(MPInP_bsInInfoSyn)
  LKAMP_bsLKAInPInfo/1 -> Switching Condition (SwtCon)/2(SwtCon_bsLKAInPInfo), Bus Selector5/1, Motion Planning Input Processing (MPInP)/4(MPInP_bsLKAInPInfo)
  LKAMP_bsLLClb/1 -> Bus Selector3/1, LKA Motion Planning Calculation (LKAMPCal)/2(LKAMPCal_bsLKAClb)
  LKAMP_stLKAActvFlg/1 -> Switching Condition (SwtCon)/1(SwtCon_stLKAActvFlg), Motion Planning Input Processing (MPInP)/2(MPInP_stLKAActvFlg)
  Bus Selector4/1 -> Switching Condition (SwtCon)/3(SwtCon_vVehSpd)  "<ESC_VehSpd>"
  LKA Motion Planning Calculation (LKAMPCal)/1(LKAMPCal_bsLKAMPCalOut) -> Steering Wheel Angle Command Calculation (SWACmdCal)/1(SWACmdCal_bsK1K2DetOut)
  Switching Condition (SwtCon)/1(SwtCon_phiHdAgMax) -> Motion Planning Input Processing (MPInP)/3(MPInP_phiHdAgMax)
  Nominal Time Calculation (NomTCalc)/1(NomTCalc_tiNomT) -> Steering Wheel Angle Command Calculation (SWACmdCal)/3(SWACmdCal_tiNomT)
  Bus Selector1/1 -> Nominal Time Calculation (NomTCalc)/1(NomTCalc_vVehSpd)  "<ESC_VehSpd>"
  Bus Selector/1 -> Nominal Time Calculation (NomTCalc)/2(NomTCalc_vVehSpdIni)  "<MPInP_vVehSpdIni>"
  Steering Wheel Angle Command Calculation (SWACmdCal)/1(SWACmdCal_phiSWACmd) -> LKAMP_phiSWACmd/1
  Steering Wheel Angle Command Calculation (SWACmdCal)/2(SWACmdCal_tiT1) -> Saturation6/1
  Motion Planning Input Processing (MPInP)/1(MPInP_bsMPInPInfo) -> Bus Selector/1, Steering Wheel Angle Command Calculation (SWACmdCal)/2(SWACmdCal_bsLKAInPInfo), LKA Motion Planning Calculation (LKAMPCal)/1(LKAMPCal_bsLKAInPInfo)  "LKAMP_bsMPInPInfo"
  Bus Selector3/2 -> Switching Condition (SwtCon)/6(SwtCon_tiHdAgExTime_C)  "<LL_HdAgExT_C>"
  Bus Selector3/3 -> Switching Condition (SwtCon)/7(SwtCon_tiLSpdCompT_C)  "<LL_LSpdCompT_C>"

== system LKAS_AutoSave_DF_20220421_1805_SW62/LKAS/LL/LLOn/LKA/LKA SWA Limit (LKASWALim) ==
  LKASWALim_phiTFCSWACmd : Inport
  LKASWALim_Ff : Inport  Port=2
  LKASWALim_bsLKAInPInfo : Inport  Port=3
  LKASWALim_bsLKAClb : Inport  Port=4
  Add : Sum  Inputs=+-+  OutDataTypeStr=single
  Add1 : Sum
  Add2 : Sum
  Bus Selector1 : BusSelector  OutputSignals=phiSWAPos,bsUndrLimInfo.UndrLim_phiSWAMax,bsUndrLimInfo.UndrLim_dphiSWARMax
  Bus Selector3 : BusSelector  OutputSignals=bsLKAClb.LL_CompSWA_C
  Gain1 : Gain  Gain=-1.4  OutDataTypeStr=single
  Gain2 : Gain  Gain=-1  OutDataTypeStr=single
  Gain3 : Gain  Gain=1.4  OutDataTypeStr=single
  "Rate Limiter Dynamic " : Subsystem
  Saturation Dynamic : simulink/Discontinuities/Saturation Dynamic  OutMin=[]  OutMax=[]  OutDataTypeStr=Inherit: Same as second input  OutDataType=fixdt(1, 16)  OutScaling=2^-10  DoSatur=off
  LKASWALim_phiSWACmd : Outport
  wires:
  Add2/1 -> Saturation Dynamic/3
  Add1/1 -> Saturation Dynamic/1
  LKASWALim_Ff/1 -> Add1/1, Add2/1
  Bus Selector1/1 -> Add/3  "<phiSWAPos>"
  LKASWALim_bsLKAInPInfo/1 -> Bus Selector1/1
  Add/1 -> Saturation Dynamic/2
  Gain1/1 -> "Rate Limiter Dynamic "/3(lo)
  Gain2/1 -> Add2/2
  Bus Selector1/3 -> Gain1/1, Gain3/1  "<UndrLim_dphiSWARMax>"
  Bus Selector1/2 -> Gain2/1, Add1/2  "<UndrLim_phiSWAMax>"
  LKASWALim_bsLKAClb/1 -> Bus Selector3/1
  LKASWALim_phiTFCSWACmd/1 -> Add/1
  Bus Selector3/1 -> Add/2  "<LL_CompSWA_C>"
  "Rate Limiter Dynamic "/1(Y) -> LKASWALim_phiSWACmd/1
  Saturation Dynamic/1 -> "Rate Limiter Dynamic "/2(u)
  Gain3/1 -> "Rate Limiter Dynamic "/1(up)

== system LKAS_AutoSave_DF_20220421_1805_SW62/LKAS/LL/LLOn/LKA/LKA_Mon ==
  BusLKA : BusCreator  Inputs=3
  CastLKA1 : DataTypeConversion  OutDataTypeStr=single
  CastLKA2 : DataTypeConversion  OutDataTypeStr=single
  CastLKA3 : DataTypeConversion  OutDataTypeStr=single
  LKAMon : Outport
  wires:
  BusLKA/1 -> LKAMon/1  "LKAMon"
  CastLKA3/1 -> BusLKA/3  "T1_Mon"
  CastLKA2/1 -> BusLKA/2  "LKA_SampleTime_Mon"
  CastLKA1/1 -> BusLKA/1  "LKA_ExitFlg_Mon"
  [T1_Mon] -> CastLKA3/1
  [LKA_SampleTime_Mon] -> CastLKA2/1
  [LKA_ExitFlg_Mon] -> CastLKA1/1

== system LKAS_AutoSave_DF_20220421_1805_SW62/LKAS/LL/LLOn/LKA/Lane Following (LF) ==
  LF_bsInInfoSyn : Inport
  LF_bsLKAInPInfo : Inport  Port=2
  LF_bsLFClb : Inport  Port=3
  Preview Information Calculation (PIC) : Subsystem  Description=|
      | Block Name:Preview Information Calculation
      | Ab.: PIC
      | No.: 02.01
      | Rev: 00.00.01
      | Update Date: 19-3-28
  Trajectory Following Control (TFC) : Subsystem  Description=|
      | Block Name:Trajectory Following Control
      | Ab.: TFC
      | No.: 02.02
      | Rev: 00.00.01
      | Update Date: 19-3-28
  LF_phiFfLFSWACmd : Outport
  LF_phiPropSWACmd : Outport  Port=2
  LF_phiIntegSWACmd : Outport  Port=3
  LF_phiDiffSWACmd : Outport  Port=4
  wires:
  LF_bsLKAInPInfo/1 -> Preview Information Calculation (PIC)/1(PIC_bsLKAInPInfo)
  Trajectory Following Control (TFC)/1(TFC_phiFfSWACmd) -> LF_phiFfLFSWACmd/1
  LF_bsInInfoSyn/1 -> Trajectory Following Control (TFC)/2(TFC_bsInInfoSyn)
  Preview Information Calculation (PIC)/1(PIC_bsPrvwInfo) -> Trajectory Following Control (TFC)/1(TFC_bsPrvwInfo)
  LF_bsLFClb/1 -> Trajectory Following Control (TFC)/3(TFC_bsTFCClb)
  Trajectory Following Control (TFC)/2(TFC_phiPropSWACmd) -> LF_phiPropSWACmd/1
  Trajectory Following Control (TFC)/3(TFC_phiIntegSWACmd) -> LF_phiIntegSWACmd/1
  Trajectory Following Control (TFC)/4(TFC_phiDiffSWACmd) -> LF_phiDiffSWACmd/1

== system LKAS_AutoSave_DF_20220421_1805_SW62/LKAS/LL/LLOn/LKA/Plan To LaneFollowing (PTLF) ==
  InP : Inport
  Plan : Inport  Port=2
  T1 : Inport  Port=3
  DrvTrq : Inport  Port=4
  Ff : Inport  Port=5
  P : Inport  Port=6
  I : Inport  Port=7
  D : Inport  Port=8
  Add1 : Sum  Inputs=+-
  Add2 : Sum  Inputs=+-
  Add3 : Sum
  Add4 : Sum  Inputs=+++++
  Add5 : Sum  Inputs=+-
  Add6 : Sum
  Bus Selector1 : BusSelector  OutputSignals=bsPrCrvtInfo.crPrvwCrvt
  Bus Selector2 : BusSelector  OutputSignals=bsHdAgInfo.phiHdAg_Lft,bsHdAgInfo.phiHdAg_Rgt
  Constant1 : Constant  Value=0.1  OutDataTypeStr=single
  Constant2 : Constant  OutDataTypeStr=single
  Divide : Product  Inputs=*/
  Divide{1..2,5..7} (5 alike) : Product  Inputs=**
  Divide3 : Product  Inputs=*/
  Divide4 : Product  Inputs=*/
  InsideJudge : Subsystem
  InsideJudge1 : Subsystem
  LowPass : Subsystem
  Saturation : Saturate  UpperLimit=1  LowerLimit=0
      settings: AttributesFormatString="Min = %<LowerLimit>  Max = %<UpperLimit>"
  Saturation1 : Saturate  UpperLimit=1  LowerLimit=0
      settings: AttributesFormatString="Min = %<LowerLimit>  Max = %<UpperLimit>"
  Saturation2 : Saturate  UpperLimit=1  LowerLimit=0
      settings: AttributesFormatString="Min = %<LowerLimit>  Max = %<UpperLimit>"
  Saturation3 : Saturate  UpperLimit=0.004  LowerLimit=-0.004
      settings: AttributesFormatString="Min = %<LowerLimit>  Max = %<UpperLimit>"
  Saturation6 : Saturate  LowerLimit=0.2
      settings: AttributesFormatString="Min = %<LowerLimit>  Max = %<UpperLimit>"
  Switch : Switch  Criteria=u2 > Threshold
  TickTime (TTime) : Subsystem
      mask Display:
      | port_label('output', 1, 'TTime');
      | color('blue');
      | text(0.98,0.9,'VCDC Block','horizontalAlignment','right');
      | color('black');
      | text(0.5,0.55,'Tick Time','horizontalAlignment','center');
      | text(0.5,0.4,'(TTime)','horizontalAlignment','center');
  TimeGain : Subsystem
  SWACmd : Outport
  tag scope: LKA_SampleTime_Mon=global, T1_Mon=global
  wires:
  Add6/1 -> Divide7/1
  [Plan] -> Add6/1
  InsideJudge1/2(Plan_1) -> [Plan]
  [Time] -> InsideJudge1/6(Time)
  Plan/1 -> InsideJudge1/5(Plan)
  T1/1 -> InsideJudge1/4(T1)
  Bus Selector2/2 -> InsideJudge1/3(HdAgRgt)  "<phiHdAg_Rgt>"
  Bus Selector2/1 -> InsideJudge1/2(HdAgLft)  "<phiHdAg_Lft>"
  [ActFlg] -> InsideJudge1/1(Flg)
  InP/1 -> Bus Selector1/1, Bus Selector2/1
  [Time] -> Add1/1
  Add1/1 -> Divide4/1
  [TFC] -> Divide4/2
  [T1] -> Add1/2
  [TFC] -> TimeGain/3(TFC)
  [T1] -> TimeGain/2(T1)
  [Time] -> TimeGain/1(Time)
  Saturation6/1 -> [TFC]
  InsideJudge1/1(T1_1) -> Saturation6/1, [T1], [T1_Mon]
  [T1] -> Divide3/2
  [Time] -> Add2/1
  [Time] -> Divide3/1
  Switch/1 -> Add4/4  "S_Ff"
  InsideJudge/1(Out1) -> Switch/2
  [ActFlg] -> InsideJudge/1(Flg)
  TickTime (TTime)/1(Out1) -> [Time]
  TimeGain/1(Out1) -> Divide5/1
  Divide5/1 -> Switch/1, Switch/3
  Saturation3/1 -> InsideJudge/2(Crvt)
  Bus Selector1/1 -> Saturation3/1  "<crPrvwCrvt>"
  Saturation1/1 -> Divide2/2
  [TFC] -> Divide/2
  Add4/1 -> LowPass/2(u)
  Add2/1 -> Divide/1
  [T1] -> Add2/2
  Divide3/1 -> Saturation/1
  Divide/1 -> Saturation2/1
  Saturation/1 -> Divide6/2
  Constant2/1 -> Add5/1
  Saturation2/1 -> Add5/2, Divide1/1
  Divide6/1 -> Add4/5  "S_DT"
  Add5/1 -> Divide7/2
  Ff/1 -> Add6/2, Divide5/2
  D/1 -> Divide2/1
  DrvTrq/1 -> Divide6/1
  Divide7/1 -> Add4/1  "S_Plan"
  P/1 -> Add3/1
  I/1 -> Add3/2
  Add3/1 -> Divide1/2
  Divide1/1 -> Add4/2  "S_PI"
  Divide4/1 -> Saturation1/1
  Divide2/1 -> Add4/3  "S_D"
  LowPass/1(y) -> SWACmd/1  "SWACmd"
  [LKA_SampleTime] -> LowPass/3(dT), [LKA_SampleTime_Mon]
  Constant1/1 -> LowPass/1(T)

== system LKAS_AutoSave_DF_20220421_1805_SW62/LKAS/LL/LLOn/LKA Input Processing (LKAInP)/Curvature Calculation (Crvt) ==
  PrvwCrvt_bsInInfoSyn : Inport
  Add : Sum  AccumDataTypeStr=single
  Bus Creator1 : BusCreator  Inputs=3
  Bus Selector1 : BusSelector  OutputSignals=bsLaneInfo.bsL0Info.L0_C2,bsLaneInfo.bsR0Info.R0_C2
  Gain : Gain  Gain=0.5
  Crvt_bsCrvtInfo : Outport
  wires:
  Bus Creator1/1 -> Crvt_bsCrvtInfo/1
  Gain/1 -> Bus Creator1/1  "crCrvt"
  PrvwCrvt_bsInInfoSyn/1 -> Bus Selector1/1
  Bus Selector1/2 -> Add/2, Bus Creator1/3  "<R0_C2>"
  Bus Selector1/1 -> Add/1, Bus Creator1/2  "<L0_C2>"
  Add/1 -> Gain/1

== system LKAS_AutoSave_DF_20220421_1805_SW62/LKAS/LL/LLOn/LKA Input Processing (LKAInP)/Deviation Calculation (Dvt) ==
  Dvt_bsInInfoSyn : Inport
  Dvt_bsLLClb : Inport  Port=2
  Add : Sum  AccumDataTypeStr=single
  Bus Creator1 : BusCreator  Inputs=3
  Bus Selector2 : BusSelector  OutputSignals=bsLaneInfo.bsL0Info.L0_C1,bsLaneInfo.bsL0Info.L0_C0,bsLaneInfo.bsR0Info.R0_C0,bsLaneInfo.bsR0Info.R0_C1
  Gain : Gain  Gain=0.5
  Left Front Conner Deviation Calculation (LFCDvtCalc) : Subsystem
  Right Front Conner Deviation Calculation (RFCDvtCalc) : Subsystem
  Dvt_bsDvtInfo : Outport
  wires:
  Dvt_bsLLClb/1 -> Right Front Conner Deviation Calculation (RFCDvtCalc)/3(RFCDvtCalc_bsLLClb), Left Front Conner Deviation Calculation (LFCDvtCalc)/3(LFCDvtCalc_bsLLClb)
  Gain/1 -> Bus Creator1/2  "lDvt"
  Add/1 -> Gain/1
  Bus Selector2/4 -> Right Front Conner Deviation Calculation (RFCDvtCalc)/2(RFCDvtCalc_bsHdAgInfo)  "<R0_C1>"
  Right Front Conner Deviation Calculation (RFCDvtCalc)/1(DvtCalc_lRgtDvt) -> Bus Creator1/3, Add/2  "IRgtDvt"
  Left Front Conner Deviation Calculation (LFCDvtCalc)/1(DvtCalc_lLftDvt) -> Add/1, Bus Creator1/1  "ILftDvt"
  Bus Selector2/3 -> Right Front Conner Deviation Calculation (RFCDvtCalc)/1(RFCDvtCalc_lDvt)  "<R0_C0>"
  Bus Selector2/2 -> Left Front Conner Deviation Calculation (LFCDvtCalc)/2(LFCDvtCalc_lDvt)  "<L0_C0>"
  Bus Creator1/1 -> Dvt_bsDvtInfo/1
  Dvt_bsInInfoSyn/1 -> Bus Selector2/1
  Bus Selector2/1 -> Left Front Conner Deviation Calculation (LFCDvtCalc)/1(LFCDvtCalc_bsHdAgInfo)  "<L0_C1>"

== system LKAS_AutoSave_DF_20220421_1805_SW62/LKAS/LL/LLOn/LKA Input Processing (LKAInP)/Heading Angle Calculation (HdAg) ==
  note: C1+2*C2*Vx*0.1
  HdAg_bsInInfoSyn : Inport
  Add1 : Sum  OutDataTypeStr=single
  Add3 : Sum  OutDataTypeStr=single
  Add4 : Sum  OutDataTypeStr=single
  Bus Creator : BusCreator  Inputs=5
  Bus Selector : BusSelector  OutputSignals=bsLaneInfo.bsL0Info.L0_C1,bsLaneInfo.bsR0Info.R0_C1,bsLaneInfo.bsL0Info.L0_C2,bsLaneInfo.bsR0Info.R0_C2,bsVehMovInfo.ESC_VehSpd
  Constant2 : Constant  Value=0.1  OutDataTypeStr=single
  Constant3 : Constant  Value=2  OutDataTypeStr=single
  Divide{1..3,5} (4 alike) : Product  Inputs=**  OutDataTypeStr=single
  Divide4 : Product  Inputs=***  OutDataTypeStr=single
  Gain : Gain  Gain=0.5  OutDataTypeStr=single
  Gain1 : Gain  Gain=1/3.6  OutDataTypeStr=single
  HdAg_bsHdAgInfo : Outport
  wires:
  Divide4/1 -> Divide5/2, Divide3/2
  Divide5/1 -> Add1/2
  Divide3/1 -> Add3/2
  Constant2/1 -> Divide4/3
  Constant3/1 -> Divide4/2
  HdAg_bsInInfoSyn/1 -> Bus Selector/1
  Gain/1 -> Bus Creator/1  "phiHdAg"
  Bus Creator/1 -> HdAg_bsHdAgInfo/1
  Bus Selector/3 -> Divide3/1  "<L0_C2>"
  Bus Selector/4 -> Divide5/1  "<R0_C2>"
  Bus Selector/5 -> Gain1/1  "<ESC_VehSpd>"
  Add3/1 -> Divide1/1, Bus Creator/2, Add4/1  "phiHdAg_Lft"
  Bus Selector/2 -> Add1/1  "<R0_C1>"
  Bus Selector/1 -> Add3/1  "<L0_C1>"
  Add1/1 -> Divide2/1, Add4/2, Bus Creator/3  "phiHdAg_Rgt"
  Add4/1 -> Gain/1
  Gain1/1 -> Divide4/1, Divide2/2, Divide1/2
  Divide1/1 -> Bus Creator/4  "Vy_L0"
  Divide2/1 -> Bus Creator/5  "Vy_R0"

== system LKAS_AutoSave_DF_20220421_1805_SW62/LKAS/LL/LLOn/LKA Input Processing (LKAInP)/Lane Width Calculation (LW) ==
  LW_bsInInfoSyn : Inport
  Abs : Abs
  Abs1 : Abs
  Add : Sum
  Bus Selector : BusSelector  OutputSignals=bsLaneInfo.bsL0Info.L0_C0,bsLaneInfo.bsR0Info.R0_C0
  Saturation : Saturate  UpperLimit=6  LowerLimit=2
      settings: AttributesFormatString="Min = %<LowerLimit>  Max = %<UpperLimit>"
  LW_LaneWidth : Outport
  wires:
  Saturation/1 -> LW_LaneWidth/1  "LaneWidth"
  Add/1 -> Saturation/1
  Abs1/1 -> Add/2
  Abs/1 -> Add/1
  Bus Selector/2 -> Abs1/1  "<R0_C0>"
  Bus Selector/1 -> Abs/1  "<L0_C0>"
  LW_bsInInfoSyn/1 -> Bus Selector/1
